simulink model "controlador_LPV_v1"  (R2018b)
settings: Solver=FixedStepAuto  StartTime=0.0  StopTime=4000  FixedStep=T  RelTol=1e-3
undefined symbols (not defined in the file): DiscIntNeverNeededParam, sp_h3, sp_h4, sp_u, T
settings Model: Creator=tarsis  LastModifiedBy=tarsis

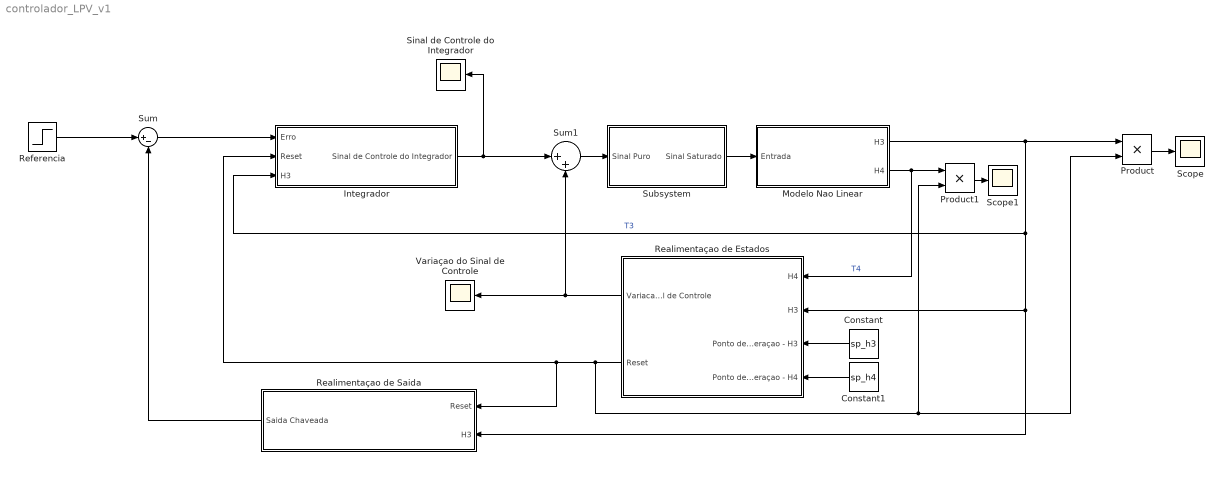
== system controlador_LPV_v1 ==
  Constant : Constant  Value=sp_h3  SampleTime=T
  Constant1 : Constant  Value=sp_h4  SampleTime=T
  Integrador : Subsystem
  Modelo Nao Linear : Subsystem
  Product : Product
  Product1 : Product
  Realimentaçao de Estados : Subsystem
  Realimentaçao de Saida : Subsystem
  Referencia : Step  Time=0  After=sp_h3  SampleTime=0
  Scope : Scope
  Scope1 : Scope
  Sinal de Controle do Integrador : Scope
  Subsystem : Subsystem
  Sum : Sum  Inputs=|+-
  Sum1 : Sum  Inputs=|++
  Variaçao do Sinal de Controle : Scope
  wires:
  Referencia/1 -> Sum/1
  Modelo Nao Linear/2(H4) -> Product1/1, Realimentaçao de Estados/1(H4)  "T4"
  Realimentaçao de Saida/1(Saida Chaveada) -> Sum/2
  Modelo Nao Linear/1(H3) -> Product/1, Integrador/3(H3), Realimentaçao de Estados/2(H3), Realimentaçao de Saida/2(H3)  "T3"
  Sum/1 -> Integrador/1(Erro)
  Constant/1 -> Realimentaçao de Estados/3(Ponto de Operaçao - H3)
  Constant1/1 -> Realimentaçao de Estados/4(Ponto de Operaçao - H4)
  Realimentaçao de Estados/1(Variacao Sinal de Controle) -> Sum1/2, Variaçao do Sinal de Controle/1
  Integrador/1(Sinal de Controle do Integrador) -> Sinal de Controle do Integrador/1, Sum1/1
  Sum1/1 -> Subsystem/1(Sinal Puro)
  Subsystem/1(Sinal Saturado) -> Modelo Nao Linear/1(Entrada)
  Product/1 -> Scope/1
  Realimentaçao de Estados/2(Reset) -> Product1/2, Product/2, Integrador/2(Reset), Realimentaçao de Saida/1(Reset)
  Product1/1 -> Scope1/1

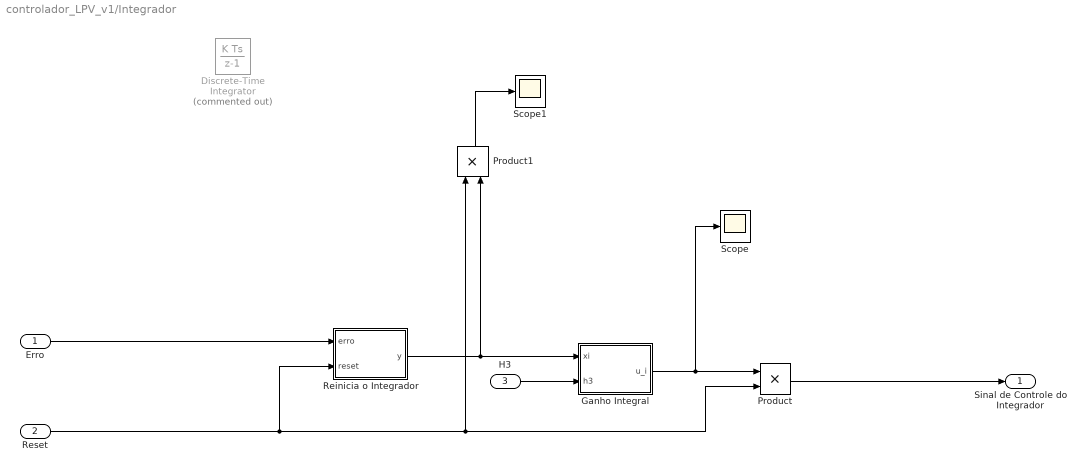
== system controlador_LPV_v1/Integrador ==
  Erro : Inport
  Reset : Inport  Port=2
  H3 : Inport  Port=3
  Discrete-Time Integrator : DiscreteIntegrator  Commented=on  gainval=1/T  ExternalReset=rising  SampleTime=T  ICPrevOutput=DiscIntNeverNeededParam  ICPrevScaledInput=DiscIntNeverNeededParam
  Ganho Integral : MATLAB Function  TreatAsAtomicUnit=on
  Product : Product
  Product1 : Product
  Reinicia o Integrador : MATLAB Function  TreatAsAtomicUnit=on  SystemSampleTime=T
  Scope : Scope
  Scope1 : Scope
  Sinal de Controle do Integrador : Outport
  wires:
  H3/1 -> Ganho Integral/2(h3)
  Reinicia o Integrador/1(y) -> Product1/2, Ganho Integral/1(xi)
  Ganho Integral/1(u_i) -> Scope/1, Product/1
  Product/1 -> Sinal de Controle do Integrador/1
  Erro/1 -> Reinicia o Integrador/1(erro)
  Product1/1 -> Scope1/1
  Reset/1 -> Reinicia o Integrador/2(reset), Product1/1, Product/2

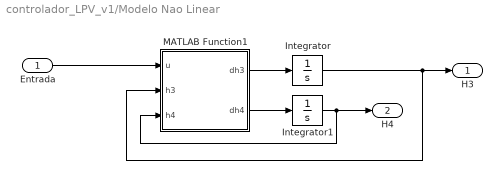
== system controlador_LPV_v1/Modelo Nao Linear ==
  Entrada : Inport
  Integrator : Integrator
  Integrator1 : Integrator
  MATLAB Function1 : MATLAB Function  TreatAsAtomicUnit=on
  H3 : Outport
  H4 : Outport  Port=2
  wires:
  Integrator1/1 -> H4/1, MATLAB Function1/3(h4)
  Entrada/1 -> MATLAB Function1/1(u)
  MATLAB Function1/2(dh4) -> Integrator1/1
  Integrator/1 -> H3/1, MATLAB Function1/2(h3)
  MATLAB Function1/1(dh3) -> Integrator/1

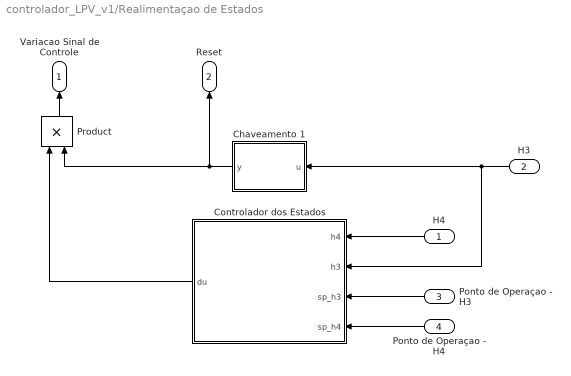
== system controlador_LPV_v1/Realimentaçao de Estados ==
  H4 : Inport
  H3 : Inport  Port=2
  Ponto de Operaçao - H3 : Inport  Port=3
  Ponto de Operaçao - H4 : Inport  Port=4
  Chaveamento 1 : MATLAB Function  TreatAsAtomicUnit=on
  Controlador dos Estados : MATLAB Function  TreatAsAtomicUnit=on  SystemSampleTime=T
  Product : Product
  Variacao Sinal de Controle : Outport
  Reset : Outport  Port=2
  wires:
  Chaveamento 1/1(y) -> Reset/1, Product/2
  H4/1 -> Controlador dos Estados/1(h4)
  H3/1 -> Chaveamento 1/1(u), Controlador dos Estados/2(h3)
  Product/1 -> Variacao Sinal de Controle/1
  Controlador dos Estados/1(du) -> Product/1
  Ponto de Operaçao - H3/1 -> Controlador dos Estados/3(sp_h3)
  Ponto de Operaçao - H4/1 -> Controlador dos Estados/4(sp_h4)

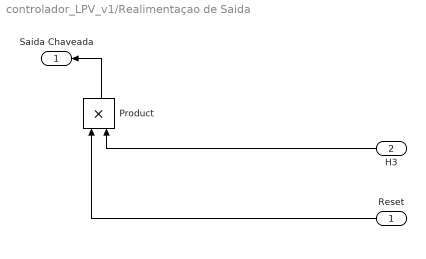
== system controlador_LPV_v1/Realimentaçao de Saida ==
  Reset : Inport
  H3 : Inport  Port=2
  Product : Product
  Saida Chaveada : Outport
  wires:
  H3/1 -> Product/2
  Product/1 -> Saida Chaveada/1
  Reset/1 -> Product/1

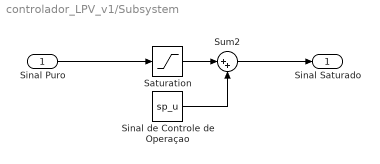
== system controlador_LPV_v1/Subsystem ==
  Sinal Puro : Inport
  Saturation : Saturate  UpperLimit=25  LowerLimit=-25
  Sinal de Controle de Operaçao : Constant  Value=sp_u  SampleTime=T
  Sum2 : Sum  Inputs=|++
  Sinal Saturado : Outport
  wires:
  Saturation/1 -> Sum2/1
  Sinal de Controle de Operaçao/1 -> Sum2/2
  Sum2/1 -> Sinal Saturado/1
  Sinal Puro/1 -> Saturation/1

== matlab function controlador_LPV_v1/Modelo Nao Linear/MATLAB Function1 ==
  data: u input; dh3 output; h3 input; h4 input; dh4 output
function [dh3,dh4] = fcn(u,h3,h4)
qi = (16.4*u + 357.3)*1e-6;
q12 = 33.51e-4*(h4 - h3) + 43.12e-5;
qout = (87.07e-5*sqrt(h3) + 30.99e-5);
A1 = (pi*(31)^2)*1e-4;
A2 = - 0.88629272879272778105782609278436*h3^16 + 6.0267905557905489111932174309337*h3^15 - 20.80464391736738395516887057851*h3^14 + 47.68494439008527766774004035511*h3^13 - 82.573907447205791291786792565001*h3^12 + 116.28257881925208875326233578017*h3^11 - 139.30893428077013388311346843447*h3^10 + 144.80767028205944702410747888441*h3^9 - 129.2475129476872169884635810807*h3^8 + 96.099152680911332924853135955618*h3^7 - 55.593870964701796673125553833866*h3^6 + 21.451550218200266654046211819752*h3^5 - 5.9275208717979510465216954484015*h3^4 + 3.9856416105248966168880953176109*h3^3 - 2.0902185091906828919771687989635*h3^2 - 0.061481774188906647716430580264178*h3 + 0.32722421068834535751546101783638;
dh4 = (qi - q12)/A1;
dh3 = (q12 - qout)/A2;

== matlab function controlador_LPV_v1/Integrador/Ganho Integral ==
  data: xi input; u_i output; h3 input
function u_i = fcn(xi,h3)
Ka1 = 719.2605;
Ka2 = 592.8033;
Ka = h3*0.05*(Ka2 - Ka1) + 2.4*Ka1 - 1.4*Ka2;
u_i = xi*Ka;

== matlab function controlador_LPV_v1/Realimentaçao de Estados/Controlador dos Estados ==
  data: h4 input; h3 input; du output; sp_h3 input; sp_h4 input
function du = fcn(h4,h3,sp_h3,sp_h4)
% Saída do Modelo não Linear
h = [h4 h3]';
% Pontos de Operação
sp_h = [sp_h4 sp_h3]';
% Ganhos do Controlador (LMI)
K1 = 1e3*[-2.4516   -4.9211];
K2 = 1e3*[-2.2695   -3.8638];
% Equação do Ganho LPV em função de alfa
K = h3*0.05*(K2 - K1) + 2.4*K1 - 1.4*K2;
% Realimentação do Estados
du = K*(h - sp_h);

== matlab function controlador_LPV_v1/Realimentaçao de Estados/Chaveamento 1 ==
  settings: updateMethod=DISCRETE
  data: u input; y output
function y = fcn(u)
persistent d
if isempty(d)
    d = true;
end

if u<0.95*0.28 && d==true
    y = 0;
else
    d = false;
    y = 1;
end

== matlab function controlador_LPV_v1/Integrador/Reinicia o Integrador ==
  settings: updateMethod=DISCRETE
  data: erro input; y output; reset input
function y = fcn(erro,reset)
% Estado do integrador
persistent xi
% Variável do Reset
persistent d
% Criando variáveis persistentes
if isempty(d)
    d = true;
end
if isempty(xi)
    xi = 0;
end
% Reset do integrador
if reset == 1 && d == true
    d = false;
    xi = 0;
end
% Ação integral
xi = erro + xi;
y = xi;
